simulink model "devWeatherFromWorkspace"  (R2018b)
settings: Solver=ode45  StartTime=0.0  StopTime=365*24*3600  RelTol=1e-3  EnableMultiTasking=on
libraries: Weather_from_Workspace x1, carnot x1
settings Model: Creator=drhf  LastModifiedBy=drhf
settings DataIOCC: LimitDataPoints=on  SaveFormat=Array  SignalLoggingSaveFormat=ModelDataLogs
settings OptimizationCC: ExpressionDepthLimit=2147483647  LifeSpan=inf
settings DebuggingCC: SolverPrmCheckMsg=warning  StateNameClashWarn=warning  SFUnexpectedBacktrackingDiag=warning  SFNoUnconditionalDefaultTransitionDiag=warning  SFExecutionAtInitializationDiag=none
settings HardwareCC: ProdBitPerPointer=32  ProdBitPerSizeT=32  ProdBitPerPtrDiffT=32  ProdLargestAtomicFloat=None  ProdIntDivRoundTo=Undefined  ProdEndianess=Unspecified  ProdWordSize=32  ProdHWDeviceType=32-bit Generic
settings ModelReferenceCC: PropagateSignalLabelsOutOfModel=off
settings SFSimCC: SimUseLocalCustomCode=off
settings RTWCC: RTWUseLocalCustomCode=off
settings CodeAppCC: StateflowObjectComments=on
settings GRTTargetCC: TargetLangStandard=C89/C90 (ANSI)  GeneratePreprocessorConditionals=Disable all  CombineOutputUpdateFcns=off  GRTInterface=on
settings ConfigComp: CovMetricSettings=dw  CovHtmlReporting=on  CovSaveCumulativeToWorkspaceVar=on  CovSaveSingleToWorkspaceVar=on  CovExternalEMLEnable=off

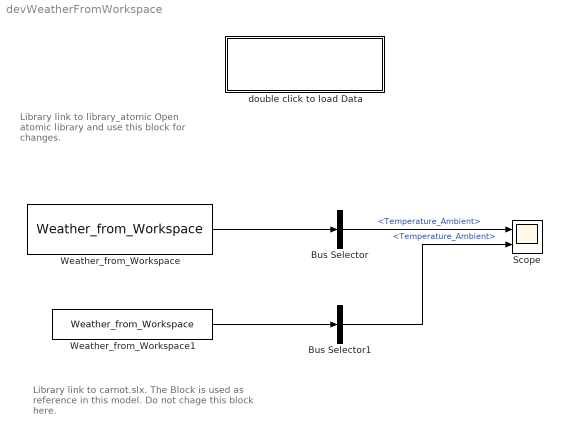
== system devWeatherFromWorkspace ==
  note: Library link to carnot.slx. The Block
      | is used as reference in this model. Do
      | not chage this block here.
  note: Library link to library_atomic
      | Open atomic library
      | and use this block for changes.
  Bus Selector : BusSelector  OutputSignals=Temperature_Ambient
  Bus Selector1 : BusSelector  OutputSignals=Temperature_Ambient
  Scope : Scope  NumInputPorts=2
  Weather_from_Workspace : Weather_from_Workspace/Weather_from_Workspace  file=DE_TRY2010_06_averageYear  SSRTWFcnClass=[]
  Weather_from_Workspace1 : carnot/Weather/Weather_from_Workspace  file=DE_TRY2010_06_averageYear
      settings: SourceProductName=Carnot
  double click to load Data : Subsystem  TreatAsAtomicUnit=on  mask{file=DE_TRY2010_06_averageYear}
      mask prompts: file "Dateiname"
      mask init:
      | %evalin('base',['load(''' file ''');'])
      | evalin('base',['datafile=(''' file ''');'])
      settings: OpenFcn=load(datafile)
      mask Display: disp(file)
  wires:
  Bus Selector/1 -> Scope/1  "<Temperature_Ambient>"
  Weather_from_Workspace/1 -> Bus Selector/1
  Weather_from_Workspace1/1 -> Bus Selector1/1
  Bus Selector1/1 -> Scope/2  "<Temperature_Ambient>"

== system devWeatherFromWorkspace/double click to load Data ==
